simulink model "test_internal_gain"  (Simulink 7.6)
settings: Solver=ode45  StartTime=0.0  StopTime=365*24*3600  RelTol=1e-3
libraries: carnot x2
settings Model: Creator=drhf  LastModifiedBy=drhf

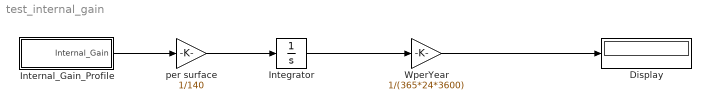
== system test_internal_gain ==
  Display : Display
  Integrator : Integrator
  Internal_Gain_Profile : Subsystem
  WperYear : Gain  Gain=1/(365*24*3600)
  per surface : Gain  Gain=1/140
  wires:
  Internal_Gain_Profile/1(Internal_Gain) -> per surface/1
  per surface/1 -> Integrator/1
  Integrator/1 -> WperYear/1
  WperYear/1 -> Display/1

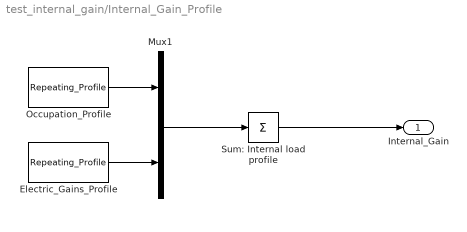
== system test_internal_gain/Internal_Gain_Profile ==
  Electric_Gains_Profile : carnot/Load/General/Repeating_Profile  SystemSampleTime=-1  period=24*3600  rep_seq_t=[0 1 6 7 8 9 11 12 13 18 19 20 22 23]*3600  rep_seq_d=[1 5 1 1 1 2 1 1 4 2 1 2 1 1]*3600  rep_seq_y=[105 55 392.5 457.5 420 55 250 55 120 170 615 420 442.5 355]
  Mux1 : Mux  Inputs=2
  Occupation_Profile : carnot/Load/General/Repeating_Profile  SystemSampleTime=-1  period=24*3600  rep_seq_t=[0 6 7 8 9 11 12 13 14 15 17 18 20 21 22]*3600  rep_seq_d=[6 1 1 1 2 1 1 1 1 2 1 2 1 1 2]*3600  rep_seq_y=[4 2 3 2 0 1 3 2 1 0 1 2 4 3 4]*60
  Sum: Internal load profile : Sum  Inputs=+
  Internal_Gain : Outport
  wires:
  Sum: Internal load profile/1 -> Internal_Gain/1
  Electric_Gains_Profile/1 -> Mux1/2
  Occupation_Profile/1 -> Mux1/1
  Mux1/1 -> Sum: Internal load profile/1
